simulink model "modelprint"  (R2023a)
settings: Solver=VariableStepAuto  StartTime=0.0  StopTime=10.0  RelTol=1e-3
values from neighbouring files (symbols this model uses):
  A_aa_disc = disc_a(1:1, 1:1)    [observer_design.m]
  A_ab_disc = disc_a(1:1, 2:4)    [observer_design.m]
  A_ba_disc = disc_a(2:4, 1:1)    [observer_design.m]
  A_bb_disc = disc_a(2:4, 2:4)    [observer_design.m]
  B_a_disc = disc_b(1:1, :)    [observer_design.m]
  B_b_disc = disc_b(2:4, :)    [observer_design.m]
  disc_sinusoid_ss = c2d(sinusoid_ss, min_sampling_time, "zoh")    [sinusoid.m]
  K_sin_int = K_sin(3)    [sinusoid.m]
  K_sin_s = K_sin(1:2)    [sinusoid.m]
  K_sin_x = K_sin(4:7)    [sinusoid.m]
  L_r_disc = place(A_bb_disc', A_ab_disc', disc_poles)'    [observer_design.m]
  w = 2 * pi / PERIOD    (= 1.57079632679)    [plotSinusoidFigure.m]    (also in sinusoid.m)
  x1_bar = deg2rad(31.78)    [reduced_order.m]
  x2_bar = deg2rad(30)    [reduced_order.m]
undefined symbols (not defined in the file or in its folder): C_l, g, I_noload, init, K_m, l, m, min_sampling_time, potentiometer_linearity_percent, R
settings Model: Creator=yunzh  LastModifiedBy=yunzh

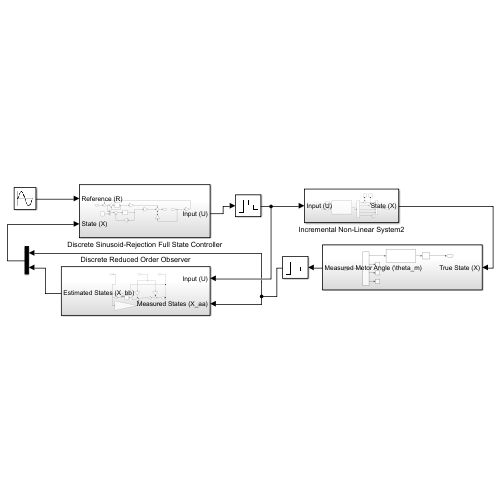
[thumbnail: Simulink's stored preview of the top-level diagram]
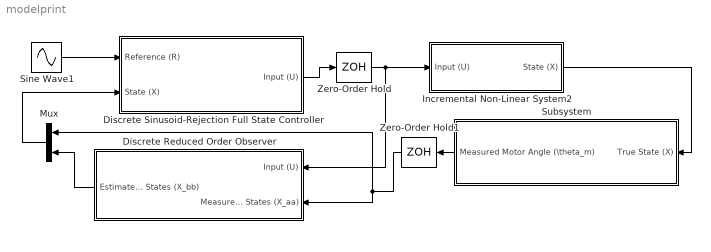
== system modelprint ==
  Discrete Reduced Order Observer : Subsystem
  Discrete Sinusoid-Rejection Full State Controller : Subsystem
  Incremental Non-Linear System2 : Subsystem
  Mux : Mux  Inputs=2
  Sine Wave1 : Sin  Amplitude=deg2rad(25)  Bias=deg2rad(-5)  Frequency=w  SampleTime=0
  Subsystem : Subsystem
  Zero-Order Hold : ZeroOrderHold  SampleTime=min_sampling_time
  Zero-Order Hold1 : ZeroOrderHold  SampleTime=min_sampling_time
  wires:
  Discrete Reduced Order Observer/1(Estimated States (X_bb)) -> Mux/2
  Sine Wave1/1 -> Discrete Sinusoid-Rejection Full State Controller/1(Reference (R))
  Discrete Sinusoid-Rejection Full State Controller/1(Input (U)) -> Zero-Order Hold/1
  Incremental Non-Linear System2/1(State (X)) -> Subsystem/1(True State (X))
  Zero-Order Hold/1 -> Incremental Non-Linear System2/1(Input (U)), Discrete Reduced Order Observer/1(Input (U))
  Mux/1 -> Discrete Sinusoid-Rejection Full State Controller/2(State (X))
  Zero-Order Hold1/1 -> Mux/1, Discrete Reduced Order Observer/2(Measured States (X_aa))
  Subsystem/1(Measured Motor Angle (\theta_m)) -> Zero-Order Hold1/1

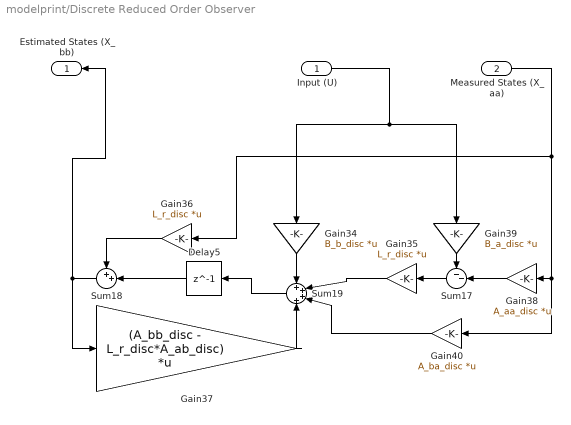
== system modelprint/Discrete Reduced Order Observer ==
  Input (U) : Inport
  Measured States (X_aa) : Inport  Port=2
  Delay5 : Delay  DelayLength=1  SampleTime=min_sampling_time
  Gain34 : Gain  Gain=B_b_disc  Multiplication=Matrix(K*u)
  Gain35 : Gain  Gain=L_r_disc  Multiplication=Matrix(K*u)
  Gain36 : Gain  Gain=L_r_disc  Multiplication=Matrix(K*u)
  Gain37 : Gain  Gain=(A_bb_disc - L_r_disc*A_ab_disc)  Multiplication=Matrix(K*u)
  Gain38 : Gain  Gain=A_aa_disc  Multiplication=Matrix(K*u)
  Gain39 : Gain  Gain=B_a_disc  Multiplication=Matrix(K*u)
  Gain40 : Gain  Gain=A_ba_disc  Multiplication=Matrix(K*u)
  Sum17 : Sum  Inputs=--|
  Sum18 : Sum  Inputs=++|
  Sum19 : Sum  Inputs=++++
  Estimated States (X_bb) : Outport
  wires:
  Gain40/1 -> Sum19/3
  Gain35/1 -> Sum19/2
  Gain37/1 -> Sum19/4
  Measured States (X_aa)/1 -> Gain38/1, Gain40/1, Gain36/1
  Gain34/1 -> Sum19/1
  Delay5/1 -> Sum18/2
  Sum17/1 -> Gain35/1
  Gain38/1 -> Sum17/2
  Sum19/1 -> Delay5/1
  Sum18/1 -> Estimated States (X_bb)/1, Gain37/1
  Gain36/1 -> Sum18/1
  Gain39/1 -> Sum17/1
  Input (U)/1 -> Gain39/1, Gain34/1

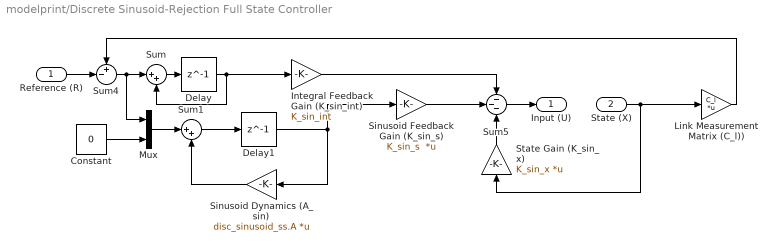
== system modelprint/Discrete Sinusoid-Rejection Full State Controller ==
  Reference (R) : Inport
  State (X) : Inport  Port=2
  Constant : Constant  Value=0
  Delay : Delay  DelayLength=1  SampleTime=min_sampling_time
  Delay1 : Delay  DelayLength=1  SampleTime=min_sampling_time
  Integral Feedback Gain (K_sin_int) : Gain  Gain=K_sin_int
  Link Measurement Matrix (C_l)) : Gain  Gain=C_l  Multiplication=Matrix(K*u)
  Mux : Mux  Inputs=2
  Sinusoid Dynamics (A_sin) : Gain  Gain=disc_sinusoid_ss.A  Multiplication=Matrix(K*u)
  Sinusoid Feedback Gain (K_sin_s) : Gain  Gain=K_sin_s  Multiplication=Matrix(K*u)
  State Gain (K_sin_x) : Gain  Gain=K_sin_x  Multiplication=Matrix(K*u)
  Sum : Sum  Inputs=|++
  Sum1 : Sum  Inputs=|++
  Sum4 : Sum  Inputs=+-|
  Sum5 : Sum  Inputs=---
  Input (U) : Outport
  wires:
  Delay/1 -> Integral Feedback Gain (K_sin_int)/1, Sum/2
  Sinusoid Feedback Gain (K_sin_s)/1 -> Sum5/2
  Sum1/1 -> Delay1/1
  Delay1/1 -> Sinusoid Dynamics (A_sin)/1, Sinusoid Feedback Gain (K_sin_s)/1
  State Gain (K_sin_x)/1 -> Sum5/3
  State (X)/1 -> Link Measurement Matrix (C_l))/1, State Gain (K_sin_x)/1
  Sum5/1 -> Input (U)/1
  Reference (R)/1 -> Sum4/2
  Sinusoid Dynamics (A_sin)/1 -> Sum1/2
  Mux/1 -> Sum1/1
  Constant/1 -> Mux/2
  Sum4/1 -> Sum/1, Mux/1
  Sum/1 -> Delay/1
  Integral Feedback Gain (K_sin_int)/1 -> Sum5/1
  Link Measurement Matrix (C_l))/1 -> Sum4/1

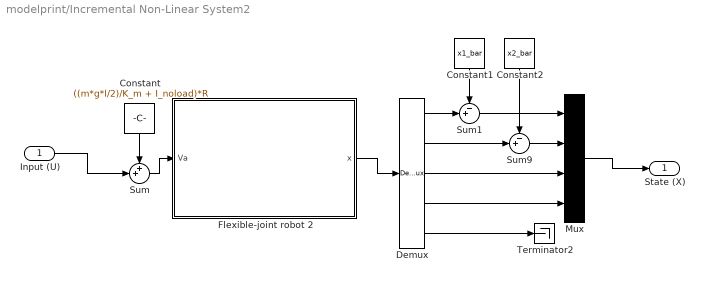
== system modelprint/Incremental Non-Linear System2 ==
  Input (U) : Inport
  Constant : Constant  Value=((m*g*l/2)/K_m + I_noload)*R
  Constant1 : Constant  Value=x1_bar
  Constant2 : Constant  Value=x2_bar
  Demux : Demux  Outputs=5
  Flexible-joint robot 2 : Subsystem
      mask Display: image('$imagefile'); % Use "Edit Image" on toolstrip to change.
  Mux : Mux
  Sum : Sum  Inputs=++|
  Sum1 : Sum  Inputs=-+|
  Sum9 : Sum  Inputs=-+|
  Terminator2 : Terminator
  State (X) : Outport
  wires:
  Flexible-joint robot 2/1(x) -> Demux/1
  Demux/1 -> Sum1/2
  Demux/2 -> Sum9/2
  Demux/5 -> Terminator2/1
  Sum/1 -> Flexible-joint robot 2/1(Va)
  Constant1/1 -> Sum1/1
  Sum9/1 -> Mux/2
  Constant2/1 -> Sum9/1
  Sum1/1 -> Mux/1
  Demux/4 -> Mux/4
  Demux/3 -> Mux/3
  Constant/1 -> Sum/1
  Input (U)/1 -> Sum/2
  Mux/1 -> State (X)/1

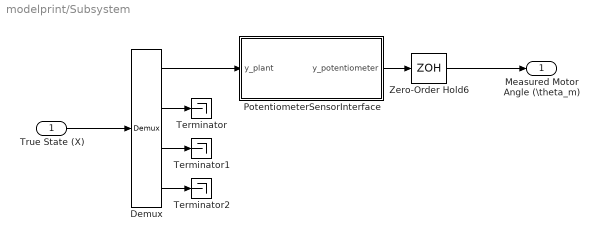
== system modelprint/Subsystem ==
  True State (X) : Inport
  Demux : Demux
  PotentiometerSensorInterface : Subsystem  TreatAsAtomicUnit=on
      mask Display: image('$imagefile'); % Use "Edit Image" on toolstrip to change.
  Terminator : Terminator
  Terminator1 : Terminator
  Terminator2 : Terminator
  Zero-Order Hold6 : ZeroOrderHold  SampleTime=min_sampling_time
  Measured Motor Angle (\theta_m) : Outport
  wires:
  PotentiometerSensorInterface/1(y_potentiometer) -> Zero-Order Hold6/1
  Demux/1 -> PotentiometerSensorInterface/1(y_plant)
  True State (X)/1 -> Demux/1
  Demux/2 -> Terminator/1
  Demux/3 -> Terminator1/1
  Demux/4 -> Terminator2/1
  Zero-Order Hold6/1 -> Measured Motor Angle (\theta_m)/1

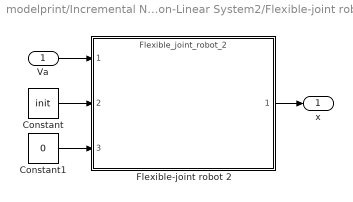
== system modelprint/Incremental Non-Linear System2/Flexible-joint robot 2 ==
  Va : Inport
  Constant : Constant  Value=init
  Constant1 : Constant  Value=0
  Flexible-joint robot 2 : ModelReference  ModelNameDialog=Flexible_joint_robot_2  ModelReferenceVersion=1.65  CopyOfModelProtected=on
  x : Outport
  wires:
  Va/1 -> Flexible-joint robot 2/1
  Constant1/1 -> Flexible-joint robot 2/3
  Constant/1 -> Flexible-joint robot 2/2
  Flexible-joint robot 2/1 -> x/1

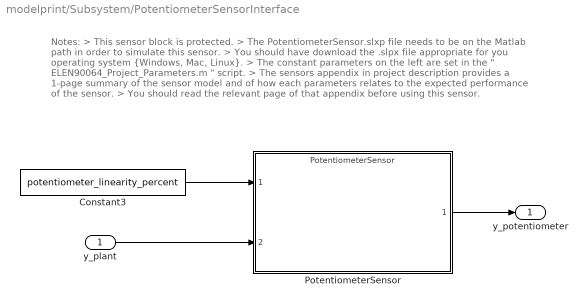
== system modelprint/Subsystem/PotentiometerSensorInterface ==
  note: Notes:
      | > This sensor block is protected.
      | > The PotentiometerSensor.slxp file needs to be on the Matlab path in order to simulate this sensor.
      | > You should have download the .slpx file appropriate for you operating system {Windows, Mac, Linux}.
      | > The constant parameters on the left are set in the " ELEN90064_Project_Parameters.m " script.
      | > The sensors appendix in project description provides a 1-page summary of the sensor model and of how each parameters relates to the expected performance of the sensor.
      | > You should read the relevant page of that appendix before using this sensor.
  y_plant : Inport
  Constant3 : Constant  Value=potentiometer_linearity_percent
  PotentiometerSensor : ModelReference  ModelNameDialog=PotentiometerSensor.slxp  ModelReferenceVersion=1.21  CopyOfModelProtected=on
  y_potentiometer : Outport
  wires:
  y_plant/1 -> PotentiometerSensor/2
  Constant3/1 -> PotentiometerSensor/1
  PotentiometerSensor/1 -> y_potentiometer/1
